simulink model "Question_5_SL"  (R2017a)
settings: Solver=VariableStepAuto  StartTime=0.0  StopTime=7  RelTol=1e-3
settings Model: PauseTimes=20  Creator=berthj01  LastModifiedBy=vonl01

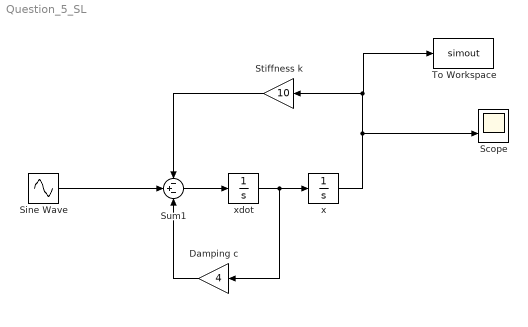
== system Question_5_SL ==
  Damping c : Gain  Gain=4
  Scope : Scope  NumInputPorts=2
  Sine Wave : Sin  Amplitude=5  Frequency=2  SampleTime=0
  Stiffness k : Gain  Gain=10
  Sum1 : Sum  Inputs=-+-
  To Workspace : ToWorkspace  VariableName=simout  SampleTime=-1
  x : Integrator  InitialCondition=1
  xdot : Integrator  InitialCondition=.5
  wires:
  xdot/1 -> Damping c/1, x/1
  Sum1/1 -> xdot/1
  Damping c/1 -> Sum1/3
  Sine Wave/1 -> Sum1/2
  Stiffness k/1 -> Sum1/1
  x/1 -> Scope/2, To Workspace/1, Stiffness k/1
